simulink model "systolicArrayFinal"  (R2021a)
settings: Solver=VariableStepAuto  StartTime=0.0  StopTime=13  RelTol=1e-3
libraries: hdlBasic x120, xbsIndex_r4 x1
(part 2 of 2)

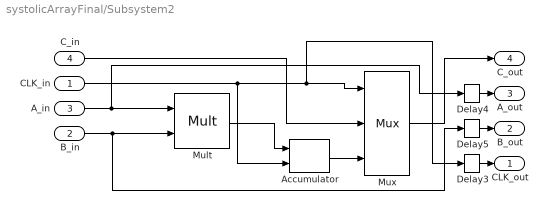
== system systolicArrayFinal/Subsystem2 ==
  CLK_in : Inport
  B_in : Inport  Port=2
  A_in : Inport  Port=3
  C_in : Inport  Port=4
  Accumulator : hdlBasic/Accumulator  operation=Add  n_bits=8  overflow=Wrap  scale=1  rst=on  hasbypass=off  en=off  latency=1  msb_inp=100  msb=100  lsb=-100  use_behavioral_HDL=on  implementation=Fabric  XmcBlockStatus=1  maskContainerNames=group3  block_type=accum  block_config=sysgen:Accum_config
  Delay3 : hdlBasic/Delay  rst=off  en=off  latency=1  reg_retiming=off  XmcBlockStatus=1  maskContainerNames=group1  block_type=delay  block_config=sysgen:Delay_config
  Delay4 : hdlBasic/Delay  rst=off  en=off  latency=1  reg_retiming=off  XmcBlockStatus=1  maskContainerNames=group1  block_type=delay  block_config=sysgen:Delay_config
  Delay5 : hdlBasic/Delay  rst=off  en=off  latency=1  reg_retiming=off  XmcBlockStatus=1  maskContainerNames=group1  block_type=delay  block_config=sysgen:Delay_config
  Mult : hdlBasic/Mult  precision=Full  arith_type="Signed  (2's comp)"  n_bits=16  bin_pt=14  quantization=Truncate  overflow=Wrap  en=off  latency=0  use_behavioral_HDL=off  opt=Speed  use_embedded=on  optimum_pipeline=off  pipeline=on  use_rpm=on  placement_style=Triangular  XmcBlockStatus=1  maskContainerNames=group1  block_type=mult  block_config=sysgen:Mult_config
  Mux : hdlBasic/Mux  inputs=2  en=off  latency=0  precision=Full  arith_type=Unsigned  n_bits=16  bin_pt=14  quantization=Truncate  overflow=Wrap  XmcBlockStatus=1  maskContainerNames=tabcontainer1  block_type=mux  block_config=sysgen:Mux_config
  CLK_out : Outport
  B_out : Outport  Port=2
  A_out : Outport  Port=3
  C_out : Outport  Port=4
  wires:
  Accumulator/1 -> Mux/3
  Mult/1 -> Accumulator/1
  Mux/1 -> C_out/1
  CLK_in/1 -> Accumulator/2, Delay3/1, Mux/1
  C_in/1 -> Mux/2
  A_in/1 -> Delay4/1, Mult/1
  B_in/1 -> Delay5/1, Mult/2
  Delay3/1 -> CLK_out/1
  Delay4/1 -> A_out/1
  Delay5/1 -> B_out/1

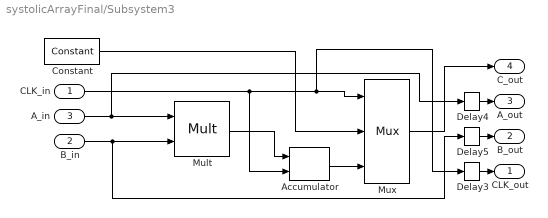
== system systolicArrayFinal/Subsystem3 ==
  CLK_in : Inport
  B_in : Inport  Port=2
  A_in : Inport  Port=3
  Accumulator : hdlBasic/Accumulator  operation=Add  n_bits=16  overflow=Wrap  scale=1  rst=on  hasbypass=off  en=off  latency=1  msb_inp=100  msb=100  lsb=-100  use_behavioral_HDL=on  implementation=Fabric  XmcBlockStatus=1  maskContainerNames=group3  block_type=accum  block_config=sysgen:Accum_config
  Constant : hdlBasic/Constant  const=0  gui_display_data_type=Fixed-point  arith_type=Signed (2's comp)  n_bits=16  bin_pt=0  preci_type=Single  exp_width=8  frac_width=24  explicit_period=off  period=1  XmcBlockStatus=1  maskContainerNames=tabcontainer1  block_type=constant  block_config=sysgen:Constant_config
  Delay3 : hdlBasic/Delay  rst=off  en=off  latency=1  reg_retiming=off  XmcBlockStatus=1  maskContainerNames=group1  block_type=delay  block_config=sysgen:Delay_config
  Delay4 : hdlBasic/Delay  rst=off  en=off  latency=1  reg_retiming=off  XmcBlockStatus=1  maskContainerNames=group1  block_type=delay  block_config=sysgen:Delay_config
  Delay5 : hdlBasic/Delay  rst=off  en=off  latency=1  reg_retiming=off  XmcBlockStatus=1  maskContainerNames=group1  block_type=delay  block_config=sysgen:Delay_config
  Mult : hdlBasic/Mult  precision=Full  arith_type="Signed  (2's comp)"  n_bits=16  bin_pt=14  quantization=Truncate  overflow=Wrap  en=off  latency=0  use_behavioral_HDL=off  opt=Speed  use_embedded=on  optimum_pipeline=off  pipeline=on  use_rpm=on  placement_style=Triangular  XmcBlockStatus=1  maskContainerNames=group1  block_type=mult  block_config=sysgen:Mult_config
  Mux : hdlBasic/Mux  inputs=2  en=off  latency=0  precision=Full  arith_type=Unsigned  n_bits=16  bin_pt=14  quantization=Truncate  overflow=Wrap  XmcBlockStatus=1  maskContainerNames=tabcontainer1  block_type=mux  block_config=sysgen:Mux_config
  CLK_out : Outport
  B_out : Outport  Port=2
  A_out : Outport  Port=3
  C_out : Outport  Port=4
  wires:
  Accumulator/1 -> Mux/3
  Mult/1 -> Accumulator/1
  Mux/1 -> C_out/1
  CLK_in/1 -> Accumulator/2, Delay3/1, Mux/1
  A_in/1 -> Delay4/1, Mult/1
  B_in/1 -> Delay5/1, Mult/2
  Delay3/1 -> CLK_out/1
  Delay4/1 -> A_out/1
  Delay5/1 -> B_out/1
  Constant/1 -> Mux/2

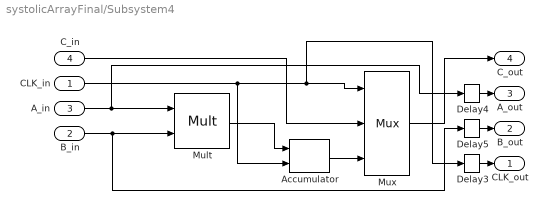
== system systolicArrayFinal/Subsystem4 ==
  CLK_in : Inport
  B_in : Inport  Port=2
  A_in : Inport  Port=3
  C_in : Inport  Port=4
  Accumulator : hdlBasic/Accumulator  operation=Add  n_bits=8  overflow=Wrap  scale=1  rst=on  hasbypass=off  en=off  latency=1  msb_inp=100  msb=100  lsb=-100  use_behavioral_HDL=on  implementation=Fabric  XmcBlockStatus=1  maskContainerNames=group3  block_type=accum  block_config=sysgen:Accum_config
  Delay3 : hdlBasic/Delay  rst=off  en=off  latency=1  reg_retiming=off  XmcBlockStatus=1  maskContainerNames=group1  block_type=delay  block_config=sysgen:Delay_config
  Delay4 : hdlBasic/Delay  rst=off  en=off  latency=1  reg_retiming=off  XmcBlockStatus=1  maskContainerNames=group1  block_type=delay  block_config=sysgen:Delay_config
  Delay5 : hdlBasic/Delay  rst=off  en=off  latency=1  reg_retiming=off  XmcBlockStatus=1  maskContainerNames=group1  block_type=delay  block_config=sysgen:Delay_config
  Mult : hdlBasic/Mult  precision=Full  arith_type="Signed  (2's comp)"  n_bits=16  bin_pt=14  quantization=Truncate  overflow=Wrap  en=off  latency=0  use_behavioral_HDL=off  opt=Speed  use_embedded=on  optimum_pipeline=off  pipeline=on  use_rpm=on  placement_style=Triangular  XmcBlockStatus=1  maskContainerNames=group1  block_type=mult  block_config=sysgen:Mult_config
  Mux : hdlBasic/Mux  inputs=2  en=off  latency=0  precision=Full  arith_type=Unsigned  n_bits=16  bin_pt=14  quantization=Truncate  overflow=Wrap  XmcBlockStatus=1  maskContainerNames=tabcontainer1  block_type=mux  block_config=sysgen:Mux_config
  CLK_out : Outport
  B_out : Outport  Port=2
  A_out : Outport  Port=3
  C_out : Outport  Port=4
  wires:
  Accumulator/1 -> Mux/3
  Mult/1 -> Accumulator/1
  Mux/1 -> C_out/1
  CLK_in/1 -> Accumulator/2, Delay3/1, Mux/1
  C_in/1 -> Mux/2
  A_in/1 -> Delay4/1, Mult/1
  B_in/1 -> Delay5/1, Mult/2
  Delay3/1 -> CLK_out/1
  Delay4/1 -> A_out/1
  Delay5/1 -> B_out/1

== system systolicArrayFinal/Subsystem5 ==
  CLK_in : Inport
  B_in : Inport  Port=2
  A_in : Inport  Port=3
  C_in : Inport  Port=4
  Accumulator : hdlBasic/Accumulator  operation=Add  n_bits=8  overflow=Wrap  scale=1  rst=on  hasbypass=off  en=off  latency=1  msb_inp=100  msb=100  lsb=-100  use_behavioral_HDL=on  implementation=Fabric  XmcBlockStatus=1  maskContainerNames=group3  block_type=accum  block_config=sysgen:Accum_config
  Delay3 : hdlBasic/Delay  rst=off  en=off  latency=1  reg_retiming=off  XmcBlockStatus=1  maskContainerNames=group1  block_type=delay  block_config=sysgen:Delay_config
  Delay4 : hdlBasic/Delay  rst=off  en=off  latency=1  reg_retiming=off  XmcBlockStatus=1  maskContainerNames=group1  block_type=delay  block_config=sysgen:Delay_config
  Delay5 : hdlBasic/Delay  rst=off  en=off  latency=1  reg_retiming=off  XmcBlockStatus=1  maskContainerNames=group1  block_type=delay  block_config=sysgen:Delay_config
  Mult : hdlBasic/Mult  precision=Full  arith_type="Signed  (2's comp)"  n_bits=16  bin_pt=14  quantization=Truncate  overflow=Wrap  en=off  latency=0  use_behavioral_HDL=off  opt=Speed  use_embedded=on  optimum_pipeline=off  pipeline=on  use_rpm=on  placement_style=Triangular  XmcBlockStatus=1  maskContainerNames=group1  block_type=mult  block_config=sysgen:Mult_config
  Mux : hdlBasic/Mux  inputs=2  en=off  latency=0  precision=Full  arith_type=Unsigned  n_bits=16  bin_pt=14  quantization=Truncate  overflow=Wrap  XmcBlockStatus=1  maskContainerNames=tabcontainer1  block_type=mux  block_config=sysgen:Mux_config
  CLK_out : Outport
  B_out : Outport  Port=2
  A_out : Outport  Port=3
  C_out : Outport  Port=4
  wires:
  Accumulator/1 -> Mux/3
  Mult/1 -> Accumulator/1
  Mux/1 -> C_out/1
  CLK_in/1 -> Accumulator/2, Delay3/1, Mux/1
  C_in/1 -> Mux/2
  A_in/1 -> Delay4/1, Mult/1
  B_in/1 -> Delay5/1, Mult/2
  Delay3/1 -> CLK_out/1
  Delay4/1 -> A_out/1
  Delay5/1 -> B_out/1

== system systolicArrayFinal/Subsystem6 ==
  CLK_in : Inport
  B_in : Inport  Port=2
  A_in : Inport  Port=3
  C_in : Inport  Port=4
  Accumulator : hdlBasic/Accumulator  operation=Add  n_bits=8  overflow=Wrap  scale=1  rst=on  hasbypass=off  en=off  latency=1  msb_inp=100  msb=100  lsb=-100  use_behavioral_HDL=on  implementation=Fabric  XmcBlockStatus=1  maskContainerNames=group3  block_type=accum  block_config=sysgen:Accum_config
  Delay3 : hdlBasic/Delay  rst=off  en=off  latency=1  reg_retiming=off  XmcBlockStatus=1  maskContainerNames=group1  block_type=delay  block_config=sysgen:Delay_config
  Delay4 : hdlBasic/Delay  rst=off  en=off  latency=1  reg_retiming=off  XmcBlockStatus=1  maskContainerNames=group1  block_type=delay  block_config=sysgen:Delay_config
  Delay5 : hdlBasic/Delay  rst=off  en=off  latency=1  reg_retiming=off  XmcBlockStatus=1  maskContainerNames=group1  block_type=delay  block_config=sysgen:Delay_config
  Mult : hdlBasic/Mult  precision=Full  arith_type="Signed  (2's comp)"  n_bits=16  bin_pt=14  quantization=Truncate  overflow=Wrap  en=off  latency=0  use_behavioral_HDL=off  opt=Speed  use_embedded=on  optimum_pipeline=off  pipeline=on  use_rpm=on  placement_style=Triangular  XmcBlockStatus=1  maskContainerNames=group1  block_type=mult  block_config=sysgen:Mult_config
  Mux : hdlBasic/Mux  inputs=2  en=off  latency=0  precision=Full  arith_type=Unsigned  n_bits=16  bin_pt=14  quantization=Truncate  overflow=Wrap  XmcBlockStatus=1  maskContainerNames=tabcontainer1  block_type=mux  block_config=sysgen:Mux_config
  CLK_out : Outport
  B_out : Outport  Port=2
  A_out : Outport  Port=3
  C_out : Outport  Port=4
  wires:
  Accumulator/1 -> Mux/3
  Mult/1 -> Accumulator/1
  Mux/1 -> C_out/1
  CLK_in/1 -> Accumulator/2, Delay3/1, Mux/1
  C_in/1 -> Mux/2
  A_in/1 -> Delay4/1, Mult/1
  B_in/1 -> Delay5/1, Mult/2
  Delay3/1 -> CLK_out/1
  Delay4/1 -> A_out/1
  Delay5/1 -> B_out/1

== system systolicArrayFinal/Subsystem7 ==
  CLK_in : Inport
  B_in : Inport  Port=2
  A_in : Inport  Port=3
  C_in : Inport  Port=4
  Accumulator : hdlBasic/Accumulator  operation=Add  n_bits=8  overflow=Wrap  scale=1  rst=on  hasbypass=off  en=off  latency=1  msb_inp=100  msb=100  lsb=-100  use_behavioral_HDL=on  implementation=Fabric  XmcBlockStatus=1  maskContainerNames=group3  block_type=accum  block_config=sysgen:Accum_config
  Delay3 : hdlBasic/Delay  rst=off  en=off  latency=1  reg_retiming=off  XmcBlockStatus=1  maskContainerNames=group1  block_type=delay  block_config=sysgen:Delay_config
  Delay4 : hdlBasic/Delay  rst=off  en=off  latency=1  reg_retiming=off  XmcBlockStatus=1  maskContainerNames=group1  block_type=delay  block_config=sysgen:Delay_config
  Delay5 : hdlBasic/Delay  rst=off  en=off  latency=1  reg_retiming=off  XmcBlockStatus=1  maskContainerNames=group1  block_type=delay  block_config=sysgen:Delay_config
  Mult : hdlBasic/Mult  precision=Full  arith_type="Signed  (2's comp)"  n_bits=16  bin_pt=14  quantization=Truncate  overflow=Wrap  en=off  latency=0  use_behavioral_HDL=off  opt=Speed  use_embedded=on  optimum_pipeline=off  pipeline=on  use_rpm=on  placement_style=Triangular  XmcBlockStatus=1  maskContainerNames=group1  block_type=mult  block_config=sysgen:Mult_config
  Mux : hdlBasic/Mux  inputs=2  en=off  latency=0  precision=Full  arith_type=Unsigned  n_bits=16  bin_pt=14  quantization=Truncate  overflow=Wrap  XmcBlockStatus=1  maskContainerNames=tabcontainer1  block_type=mux  block_config=sysgen:Mux_config
  CLK_out : Outport
  B_out : Outport  Port=2
  A_out : Outport  Port=3
  C_out : Outport  Port=4
  wires:
  Accumulator/1 -> Mux/3
  Mult/1 -> Accumulator/1
  Mux/1 -> C_out/1
  CLK_in/1 -> Accumulator/2, Delay3/1, Mux/1
  C_in/1 -> Mux/2
  A_in/1 -> Delay4/1, Mult/1
  B_in/1 -> Delay5/1, Mult/2
  Delay3/1 -> CLK_out/1
  Delay4/1 -> A_out/1
  Delay5/1 -> B_out/1

== system systolicArrayFinal/Subsystem8 ==
  CLK_in : Inport
  B_in : Inport  Port=2
  A_in : Inport  Port=3
  C_in : Inport  Port=4
  Accumulator : hdlBasic/Accumulator  operation=Add  n_bits=8  overflow=Wrap  scale=1  rst=on  hasbypass=off  en=off  latency=1  msb_inp=100  msb=100  lsb=-100  use_behavioral_HDL=on  implementation=Fabric  XmcBlockStatus=1  maskContainerNames=group3  block_type=accum  block_config=sysgen:Accum_config
  Delay3 : hdlBasic/Delay  rst=off  en=off  latency=1  reg_retiming=off  XmcBlockStatus=1  maskContainerNames=group1  block_type=delay  block_config=sysgen:Delay_config
  Delay4 : hdlBasic/Delay  rst=off  en=off  latency=1  reg_retiming=off  XmcBlockStatus=1  maskContainerNames=group1  block_type=delay  block_config=sysgen:Delay_config
  Delay5 : hdlBasic/Delay  rst=off  en=off  latency=1  reg_retiming=off  XmcBlockStatus=1  maskContainerNames=group1  block_type=delay  block_config=sysgen:Delay_config
  Mult : hdlBasic/Mult  precision=Full  arith_type="Signed  (2's comp)"  n_bits=16  bin_pt=14  quantization=Truncate  overflow=Wrap  en=off  latency=0  use_behavioral_HDL=off  opt=Speed  use_embedded=on  optimum_pipeline=off  pipeline=on  use_rpm=on  placement_style=Triangular  XmcBlockStatus=1  maskContainerNames=group1  block_type=mult  block_config=sysgen:Mult_config
  Mux : hdlBasic/Mux  inputs=2  en=off  latency=0  precision=Full  arith_type=Unsigned  n_bits=16  bin_pt=14  quantization=Truncate  overflow=Wrap  XmcBlockStatus=1  maskContainerNames=tabcontainer1  block_type=mux  block_config=sysgen:Mux_config
  CLK_out : Outport
  B_out : Outport  Port=2
  A_out : Outport  Port=3
  C_out : Outport  Port=4
  wires:
  Accumulator/1 -> Mux/3
  Mult/1 -> Accumulator/1
  Mux/1 -> C_out/1
  CLK_in/1 -> Accumulator/2, Delay3/1, Mux/1
  C_in/1 -> Mux/2
  A_in/1 -> Delay4/1, Mult/1
  B_in/1 -> Delay5/1, Mult/2
  Delay3/1 -> CLK_out/1
  Delay4/1 -> A_out/1
  Delay5/1 -> B_out/1

== system systolicArrayFinal/Subsystem9 ==
  CLK_in : Inport
  B_in : Inport  Port=2
  A_in : Inport  Port=3
  C_in : Inport  Port=4
  Accumulator : hdlBasic/Accumulator  operation=Add  n_bits=8  overflow=Wrap  scale=1  rst=on  hasbypass=off  en=off  latency=1  msb_inp=100  msb=100  lsb=-100  use_behavioral_HDL=on  implementation=Fabric  XmcBlockStatus=1  maskContainerNames=group3  block_type=accum  block_config=sysgen:Accum_config
  Delay3 : hdlBasic/Delay  rst=off  en=off  latency=1  reg_retiming=off  XmcBlockStatus=1  maskContainerNames=group1  block_type=delay  block_config=sysgen:Delay_config
  Delay4 : hdlBasic/Delay  rst=off  en=off  latency=1  reg_retiming=off  XmcBlockStatus=1  maskContainerNames=group1  block_type=delay  block_config=sysgen:Delay_config
  Delay5 : hdlBasic/Delay  rst=off  en=off  latency=1  reg_retiming=off  XmcBlockStatus=1  maskContainerNames=group1  block_type=delay  block_config=sysgen:Delay_config
  Mult : hdlBasic/Mult  precision=Full  arith_type="Signed  (2's comp)"  n_bits=16  bin_pt=14  quantization=Truncate  overflow=Wrap  en=off  latency=0  use_behavioral_HDL=off  opt=Speed  use_embedded=on  optimum_pipeline=off  pipeline=on  use_rpm=on  placement_style=Triangular  XmcBlockStatus=1  maskContainerNames=group1  block_type=mult  block_config=sysgen:Mult_config
  Mux : hdlBasic/Mux  inputs=2  en=off  latency=0  precision=Full  arith_type=Unsigned  n_bits=16  bin_pt=14  quantization=Truncate  overflow=Wrap  XmcBlockStatus=1  maskContainerNames=tabcontainer1  block_type=mux  block_config=sysgen:Mux_config
  CLK_out : Outport
  B_out : Outport  Port=2
  A_out : Outport  Port=3
  C_out : Outport  Port=4
  wires:
  Accumulator/1 -> Mux/3
  Mult/1 -> Accumulator/1
  Mux/1 -> C_out/1
  CLK_in/1 -> Accumulator/2, Delay3/1, Mux/1
  C_in/1 -> Mux/2
  A_in/1 -> Delay4/1, Mult/1
  B_in/1 -> Delay5/1, Mult/2
  Delay3/1 -> CLK_out/1
  Delay4/1 -> A_out/1
  Delay5/1 -> B_out/1
